simulink model "chap9_3sim"  (Simulink 8.1)
settings: Solver=ode45  StartTime=0.0  StopTime=30  FixedStep=0.005  RelTol=1e-3
settings Model: Creator=hp  LastModifiedBy=liujk  ExtModeTrigMode=oneshot  ExtModeArmWhenConnect=off
settings DataIOCC: LimitDataPoints=off  SignalLoggingName=sigsOut
settings OptimizationCC: BooleanDataType=off  InitFltsAndDblsToZero=on
settings DebuggingCC: SaveWithParameterizedLinksMsg=none  SignalResolutionControl=TryResolveAllWithWarning  SolverPrmCheckMsg=none  MultiTaskDSMMsg=warning  MultiTaskCondExecSysMsg=none  StrictBusMsg=None
settings HardwareCC: TargetUnknown=on
settings RTWCC: IncludeERTFirstTime=on
settings GRTTargetCC: TargetFcnLib=ansi_tfl_tmw.mat

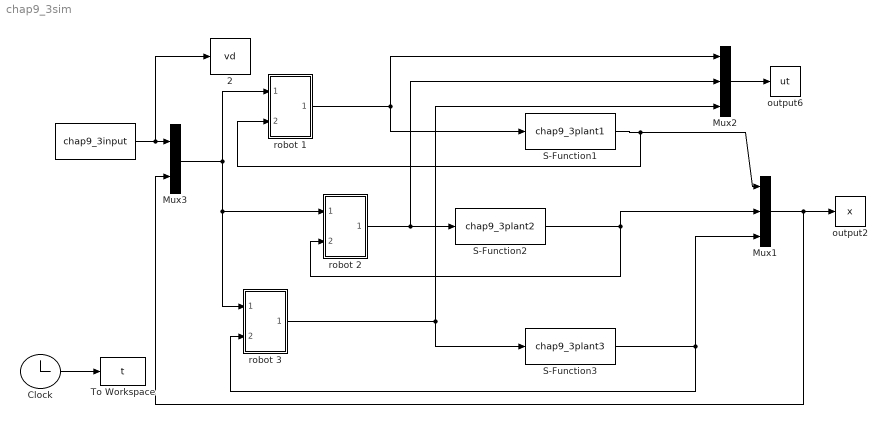
== system chap9_3sim ==
  " " : S-Function  FunctionName=chap9_3input  EnableBusSupport=off
  "   2" : ToWorkspace  VariableName=vd  SampleTime=-1
  Clock : Clock
  Mux1 : Mux  Inputs=3
  Mux2 : Mux  Inputs=3
  Mux3 : Mux  Inputs=2
  S-Function1 : S-Function  FunctionName=chap9_3plant1  EnableBusSupport=off
  S-Function2 : S-Function  FunctionName=chap9_3plant2  EnableBusSupport=off
  S-Function3 : S-Function  FunctionName=chap9_3plant3  EnableBusSupport=off
  To Workspace : ToWorkspace  VariableName=t  SampleTime=-1
  output2 : ToWorkspace  VariableName=x  SampleTime=-1
  output6 : ToWorkspace  VariableName=ut  SampleTime=-1
  robot 1 : Subsystem
  robot 2 : Subsystem
  robot 3 : Subsystem
  wires:
  Clock/1 -> To Workspace/1
  " "/1 -> "   2"/1, Mux3/1
  Mux3/1 -> robot 1/1(In1), robot 2/1(In1), robot 3/1(In1)
  robot 1/1(Out1) -> S-Function1/1, Mux2/1
  robot 2/1(Out1) -> S-Function2/1, Mux2/2
  robot 3/1(Out1) -> S-Function3/1, Mux2/3
  S-Function1/1 -> Mux1/1, robot 1/2(In2)
  S-Function2/1 -> robot 2/2(In2), Mux1/2
  S-Function3/1 -> Mux1/3, robot 3/2(In2)
  Mux1/1 -> output2/1, Mux3/2
  Mux2/1 -> output6/1

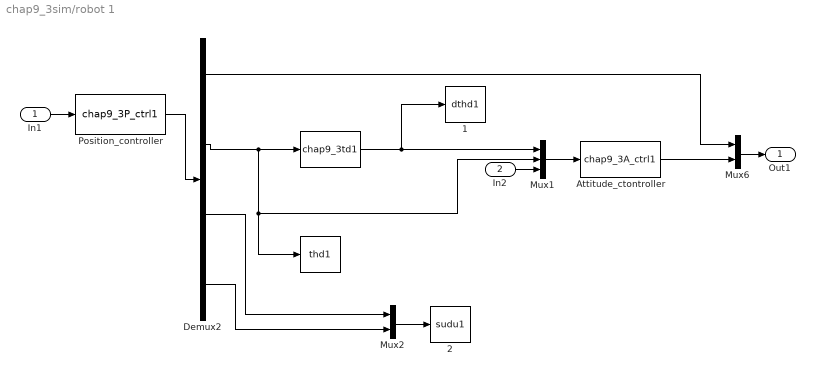
== system chap9_3sim/robot 1 ==
  In1 : Inport
  In2 : Inport  Port=2
  "  " : S-Function  FunctionName=chap9_3td1  EnableBusSupport=off
  "   " : ToWorkspace  VariableName=thd1  SampleTime=-1
  "   1" : ToWorkspace  VariableName=dthd1  SampleTime=-1
  "   2" : ToWorkspace  VariableName=sudu1  SampleTime=-1
  Attitude_ctontroller : S-Function  FunctionName=chap9_3A_ctrl1  EnableBusSupport=off
  Demux2 : Demux
  Mux1 : Mux  Inputs=3
  Mux2 : Mux  Inputs=2
  Mux6 : Mux  Inputs=2
  Position_controller : S-Function  FunctionName=chap9_3P_ctrl1  EnableBusSupport=off
  Out1 : Outport
  wires:
  Demux2/2 -> "   "/1, Mux1/2, "  "/1
  "  "/1 -> "   1"/1, Mux1/1
  Attitude_ctontroller/1 -> Mux6/2
  Position_controller/1 -> Demux2/1
  Mux1/1 -> Attitude_ctontroller/1
  Demux2/1 -> Mux6/1
  In1/1 -> Position_controller/1
  Mux6/1 -> Out1/1
  In2/1 -> Mux1/3
  Mux2/1 -> "   2"/1
  Demux2/3 -> Mux2/1
  Demux2/4 -> Mux2/2

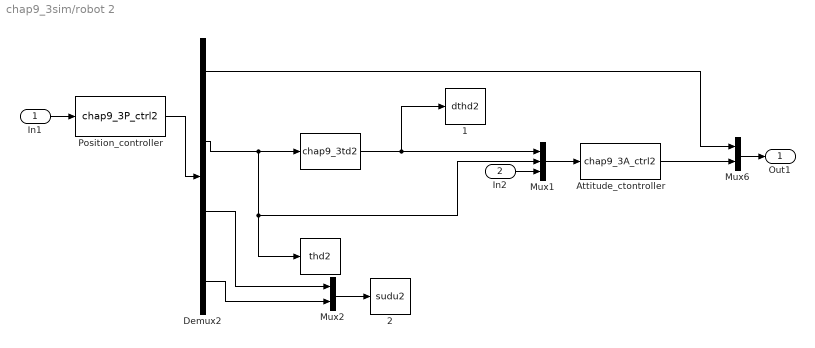
== system chap9_3sim/robot 2 ==
  In1 : Inport
  In2 : Inport  Port=2
  "  " : S-Function  FunctionName=chap9_3td2  EnableBusSupport=off
  "   " : ToWorkspace  VariableName=thd2  SampleTime=-1
  "   1" : ToWorkspace  VariableName=dthd2  SampleTime=-1
  "   2" : ToWorkspace  VariableName=sudu2  SampleTime=-1
  Attitude_ctontroller : S-Function  FunctionName=chap9_3A_ctrl2  EnableBusSupport=off
  Demux2 : Demux
  Mux1 : Mux  Inputs=3
  Mux2 : Mux  Inputs=2
  Mux6 : Mux  Inputs=2
  Position_controller : S-Function  FunctionName=chap9_3P_ctrl2  EnableBusSupport=off
  Out1 : Outport
  wires:
  Demux2/2 -> "   "/1, Mux1/2, "  "/1
  "  "/1 -> "   1"/1, Mux1/1
  Attitude_ctontroller/1 -> Mux6/2
  Position_controller/1 -> Demux2/1
  Mux1/1 -> Attitude_ctontroller/1
  Demux2/1 -> Mux6/1
  In1/1 -> Position_controller/1
  Mux6/1 -> Out1/1
  In2/1 -> Mux1/3
  Demux2/3 -> Mux2/1
  Mux2/1 -> "   2"/1
  Demux2/4 -> Mux2/2

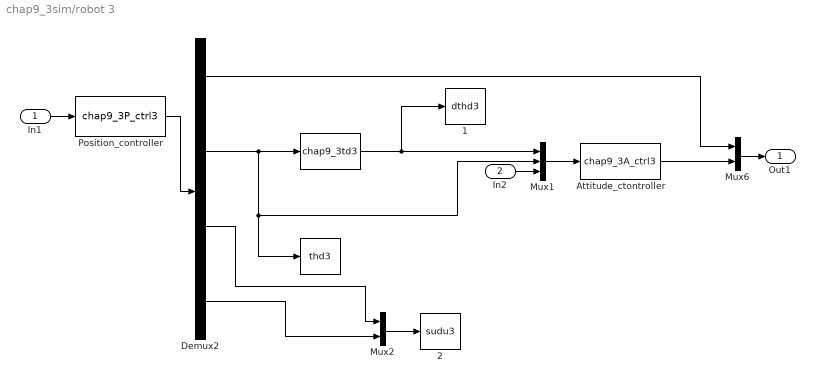
== system chap9_3sim/robot 3 ==
  In1 : Inport
  In2 : Inport  Port=2
  "  " : S-Function  FunctionName=chap9_3td3  EnableBusSupport=off
  "   " : ToWorkspace  VariableName=thd3  SampleTime=-1
  "   1" : ToWorkspace  VariableName=dthd3  SampleTime=-1
  "   2" : ToWorkspace  VariableName=sudu3  SampleTime=-1
  Attitude_ctontroller : S-Function  FunctionName=chap9_3A_ctrl3  EnableBusSupport=off
  Demux2 : Demux
  Mux1 : Mux  Inputs=3
  Mux2 : Mux  Inputs=2
  Mux6 : Mux  Inputs=2
  Position_controller : S-Function  FunctionName=chap9_3P_ctrl3  EnableBusSupport=off
  Out1 : Outport
  wires:
  Demux2/2 -> "   "/1, Mux1/2, "  "/1
  "  "/1 -> "   1"/1, Mux1/1
  Attitude_ctontroller/1 -> Mux6/2
  Position_controller/1 -> Demux2/1
  Mux1/1 -> Attitude_ctontroller/1
  Demux2/1 -> Mux6/1
  In1/1 -> Position_controller/1
  Mux6/1 -> Out1/1
  In2/1 -> Mux1/3
  Demux2/3 -> Mux2/1
  Mux2/1 -> "   2"/1
  Demux2/4 -> Mux2/2
